simulink library "lib_controls"  (Simulink 7.9)
settings: Solver=ode45  SolverMode=SingleTasking  StartTime=0.0  StopTime=10.0  RelTol=1e-3
undefined symbols (not defined in the file): amb_tmp, cs_charge_deplete_bool, cs_charge_pwr, cs_charge_trq, cs_clt_tmp, cs_decel_fc_off, cs_decel_regen_threshold, cs_dl_assist_trq_threshold, cs_dl_regen_trq_threshold, cs_electric_decel_spd, cs_electric_launch_spd, cs_electric_launch_spd_hi, cs_electric_launch_spd_lo, cs_eng_min_spd, cs_eng_on_soc, cs_fc_init_state, cs_fc_max_pwr_frac, cs_fc_min_pwr_frac, cs_fc_on, cs_fc_pwr_opt, cs_fc_spd_opt, cs_fuzzy_fuel_mode, cs_hi_soc, cs_hi_trq_frac, cs_lo_soc, cs_lo_trq_frac, cs_max_gc_spd, cs_max_pwr, cs_max_pwr_fall_rate, cs_max_pwr_rise_rate, cs_mc_assist_max_frac, cs_mc_assist_min_frac, cs_mc_assist_slope, cs_mc_regen_max_frac, cs_mc_regen_min_frac, cs_mc_regen_slope, cs_mean_eff, cs_mean_eff_bool, cs_min_gc_spd, cs_min_off_time, cs_min_pwr, cs_min_trq_frac, cs_mph_avg_time, cs_off_trq_frac, cs_plot_output, cs_pwr, cs_regen_avg_time, cs_scale_factor, cs_shutoff, cs_soc_range, cs_spd, cs_target_soc, cs_trq_to_soc_factor, cvt_locus_pwr, cvt_locus_spd, cyc_mph, enable_sim_stop_distance, enable_sim_stop_max_spd, enable_sim_stop_speed, enable_sim_stop_time ... (+110)
libraries: lib_controls x124, simulink3 x18, lib_etc x1
(part 16 of 17)

== system lib_controls/<vc> par auto/gearbox control for use w/ AT/shifting1/time since last shift ==
  in_1 : Inport
  just shifted : Subsystem
      mask Display: disp('just\nshifted')
  timer : Subsystem
      mask Display: disp('timer')
  out_1 : Outport  InitialOutput=0
  wires:
  in_1/1 -> just shifted/1(in_1)
  just shifted/1(out_1) -> timer/1(trigger)
  timer/1(time) -> out_1/1

== system lib_controls/<vc> par auto/gearbox control for use w/ AT/upshift  command/load fraction ==
  In1 : Inport
  S-Function : S-Function  FunctionName=sfun_gearbox  Parameters=load, spd  EnableBusSupport=off
  Out1 : Outport  InitialOutput=0
  wires:
  S-Function/1 -> Out1/1
  In1/1 -> S-Function/1

== system lib_controls/<vc> par auto/parallel clutch control/gearbox speed estimator/Block NOTES ==
  note: The requested engine speed is replaced by an estimate of the
      | engine's previous speed whenever the vehicle missed the trace
      |  by more than 1 mph on the last time step.

== system lib_controls/<vc> par auto/parallel clutch control/gearbox speed estimator/dt ==
  Clock : Clock
  Memory1 : Memory  X0=-1
  Sum4 : Sum  Inputs=+-  SaturateOnIntegerOverflow=on  InputSameDT=on  OutDataTypeStr=Inherit: Same as first input
  Out1 : Outport  InitialOutput=0
  wires:
  Clock/1 -> Sum4/1, Memory1/1
  Memory1/1 -> Sum4/2
  Sum4/1 -> Out1/1

== system lib_controls/<vc> par auto s/a/gearbox control for use w/ AT  in parallel sa/downshift  command/load fraction ==
  In1 : Inport
  S-Function : S-Function  FunctionName=sfun_gearbox  Parameters=load, spd  EnableBusSupport=off
  Out1 : Outport  InitialOutput=0
  wires:
  S-Function/1 -> Out1/1
  In1/1 -> S-Function/1

== system lib_controls/<vc> par auto s/a/gearbox control for use w/ AT  in parallel sa/downshift  command1/load fraction ==
  In1 : Inport
  S-Function : S-Function  FunctionName=sfun_gearbox  Parameters=load, spd  EnableBusSupport=off
  Out1 : Outport  InitialOutput=0
  wires:
  In1/1 -> S-Function/1
  S-Function/1 -> Out1/1

== system lib_controls/<vc> par auto s/a/gearbox control for use w/ AT  in parallel sa/est. engine trq and spd/Block NOTES ==
  note: Estimate engine torque and speed associated with the previous gear, assuming that
      | the gearbox efficiency is constant.

== system lib_controls/<vc> par auto s/a/gearbox control for use w/ AT  in parallel sa/est. engine trq and spd/K_adv ==
  "Req'd output trq and spd (Nm), (rad/s)" : Inport
  K_adv=wout/(Tout)^0.5 : Fcn  Expr=u[2]/u[1]^0.5
  Saturation : Saturate  UpperLimit=max(htc_k_adv)  LowerLimit=min(htc_k_adv)
  Saturation2 : Saturate  UpperLimit=inf  LowerLimit=eps
  K_adv : Outport
  wires:
  "Req'd output trq and spd (Nm), (rad/s)"/1 -> Saturation2/1
  Saturation2/1 -> K_adv=wout/(Tout)^0.5/1
  K_adv=wout/(Tout)^0.5/1 -> Saturation/1
  Saturation/1 -> K_adv/1

== system lib_controls/<vc> par auto s/a/gearbox control for use w/ AT  in parallel sa/est. engine trq and spd assuming lockup/Block NOTES ==
  note: Estimate engine torque and speed associated with the current gear, assuming that
      | the gearbox efficiency is constant.

== system lib_controls/<vc> par auto s/a/gearbox control for use w/ AT  in parallel sa/shifting1/time since last shift ==
  in_1 : Inport
  just shifted : Subsystem
      mask Display: disp('just\nshifted')
  timer : Subsystem
      mask Display: disp('timer')
  out_1 : Outport  InitialOutput=0
  wires:
  in_1/1 -> just shifted/1(in_1)
  just shifted/1(out_1) -> timer/1(trigger)
  timer/1(time) -> out_1/1

== system lib_controls/<vc> par auto s/a/gearbox control for use w/ AT  in parallel sa/upshift  command/load fraction ==
  In1 : Inport
  S-Function : S-Function  FunctionName=sfun_gearbox  Parameters=load, spd  EnableBusSupport=off
  Out1 : Outport  InitialOutput=0
  wires:
  S-Function/1 -> Out1/1
  In1/1 -> S-Function/1

== system lib_controls/<vc> par balanced/parallel clutch control/gearbox speed estimator/Block NOTES ==
  note: The requested engine speed is replaced by an estimate of the
      | engine's previous speed whenever the vehicle missed the trace
      |  by more than 1 mph on the last time step.

== system lib_controls/<vc> par balanced/parallel clutch control/gearbox speed estimator/dt ==
  Clock : Clock
  Memory1 : Memory  X0=-1
  Sum4 : Sum  Inputs=+-  SaturateOnIntegerOverflow=on  InputSameDT=on  OutDataTypeStr=Inherit: Same as first input
  Out1 : Outport  InitialOutput=0
  wires:
  Clock/1 -> Sum4/1, Memory1/1
  Memory1/1 -> Sum4/2
  Sum4/1 -> Out1/1

== system lib_controls/<vc> par balanced/pre-TX parallel gearbox control/allow upshift?/Block NOTES1 ==
  note: This block prevents an upshift if it the engine is not on and
      | the upshift would make the motor power low enough that it
      | could not provide the required input power.  However, an upshift
      | is allowed if to stay in the current gear would put the motor
      | beyond 95% of its maximum speed.
      |
      | This block is to be used in pretransmission parallel hybrids
      | (where the engine and motor torques are combined on the
      | engine side of the transmission) ONLY.

== system lib_controls/<vc> par balanced/pre-TX parallel gearbox control/downshift  command/load fraction ==
  In1 : Inport
  S-Function : S-Function  FunctionName=sfun_gearbox  Parameters=load, spd  EnableBusSupport=off
  Out1 : Outport  InitialOutput=0
  wires:
  In1/1 -> S-Function/1
  S-Function/1 -> Out1/1

== system lib_controls/<vc> par balanced/pre-TX parallel gearbox control/gearbox speed estimator/Block NOTES ==
  note: The requested engine speed is replaced by an estimate of the
      | engine's previous speed whenever the vehicle missed the trace
      |  by more than 1 mph on the last time step.

== system lib_controls/<vc> par balanced/pre-TX parallel gearbox control/gearbox speed estimator/dt ==
  Clock : Clock
  Memory1 : Memory  X0=-1
  Sum4 : Sum  Inputs=+-  SaturateOnIntegerOverflow=on  InputSameDT=on  OutDataTypeStr=Inherit: Same as first input
  Out1 : Outport  InitialOutput=0
  wires:
  Clock/1 -> Sum4/1, Memory1/1
  Memory1/1 -> Sum4/2
  Sum4/1 -> Out1/1

== system lib_controls/<vc> par balanced/pre-TX parallel gearbox control/shifting1/time since last shift ==
  in_1 : Inport
  just shifted : Subsystem
      mask Display: disp('just\nshifted')
  timer : Subsystem
      mask Display: disp('timer')
  out_1 : Outport  InitialOutput=0
  wires:
  in_1/1 -> just shifted/1(in_1)
  just shifted/1(out_1) -> timer/1(trigger)
  timer/1(time) -> out_1/1

== system lib_controls/<vc> par balanced/pre-TX parallel gearbox control/upshift  command/load fraction ==
  In1 : Inport
  S-Function : S-Function  FunctionName=sfun_gearbox  Parameters=load, spd  EnableBusSupport=off
  Out1 : Outport  InitialOutput=0
  wires:
  In1/1 -> S-Function/1
  S-Function/1 -> Out1/1

== system lib_controls/<vc> par cvt/cvt control/Mode Selector/Block NOTES ==
  note: This block determines the operating mode of the parallel
      | hybrid vehicle equipped with a CVT:
      | Mode 1: motor only regen
      | if trq request is negative
      | Mode 2: motor only driving
      | if soc is greater than lo soc
      | and
      | pwr req is less than min engine pwr frac
      | Mode3: engine primary with motor assist
      | if pwr request between min and max pwr fractions
      | or
      | if soc less than low soc
      | Mode4: engine and motor combined system
      | if pwr req greater than max engine pwr frac

== system lib_controls/<vc> par cvt/parallel clutch control/gearbox speed estimator/Block NOTES ==
  note: The requested engine speed is replaced by an estimate of the
      | engine's previous speed whenever the vehicle missed the trace
      |  by more than 1 mph on the last time step.

== system lib_controls/<vc> par cvt/parallel clutch control/gearbox speed estimator/dt ==
  Clock : Clock
  Memory1 : Memory  X0=-1
  Sum4 : Sum  Inputs=+-  SaturateOnIntegerOverflow=on  InputSameDT=on  OutDataTypeStr=Inherit: Same as first input
  Out1 : Outport  InitialOutput=0
  wires:
  Sum4/1 -> Out1/1
  Memory1/1 -> Sum4/2
  Clock/1 -> Memory1/1, Sum4/1

== system lib_controls/<vc> prius/Coordinated  Controller/max engine efficiency point/Max fc spd (rad/s) ==
  mc spd : Inport
  <fc max rpm : Saturate  UpperLimit=4000*2*pi/60  LowerLimit=0
  f(gc max spd,veh spd) : Fcn  Expr=tx_pg_r/(tx_pg_r + tx_pg_s)*u + tx_pg_s/(tx_pg_r + tx_pg_s)*cs_max_gc_spd
  Max fc spd rad/s : Outport  InitialOutput=0
  wires:
  <fc max rpm/1 -> Max fc spd rad/s/1
  mc spd/1 -> f(gc max spd,veh spd)/1
  f(gc max spd,veh spd)/1 -> <fc max rpm/1

== system lib_controls/<vc> prius/Coordinated  Controller/max engine efficiency point/Min fc spd(rad/s) ==
  mc spd : Inport
  Constant2 : Constant  Value=vc_idle_spd
  Constant3 : Constant  Value=0
  MinMax1 : MinMax  Function=max  Inputs=2  SaturateOnIntegerOverflow=on  InputSameDT=on
  Switch2 : Switch  SaturateOnIntegerOverflow=on  InputSameDT=on
  To Workspace3 : ToWorkspace  VariableName=fc_min_spd  SampleTime=-1
  f(gc max spd,veh spd) : Fcn  Expr=tx_pg_r/(tx_pg_r + tx_pg_s)*u + tx_pg_s/(tx_pg_r + tx_pg_s)*cs_min_gc_spd
  min fc spd rad/s : Outport  InitialOutput=0
  wires:
  Switch2/1 -> To Workspace3/1, min fc spd rad/s/1
  Constant3/1 -> Switch2/3
  MinMax1/1 -> Switch2/1
  Constant2/1 -> MinMax1/1
  f(gc max spd,veh spd)/1 -> Switch2/2, MinMax1/2
  mc spd/1 -> f(gc max spd,veh spd)/1

== system lib_controls/<vc> prius/Coordinated  Controller/max engine efficiency point/at least  idle speed ==
  trq : Inport
  spd : Inport  Port=2
  Constant2 : Constant  Value=vc_idle_spd
  MinMax4 : MinMax  Function=max  Inputs=2  SaturateOnIntegerOverflow=on  InputSameDT=on
  Product : Product  SaturateOnIntegerOverflow=on  RndMeth=Zero  InputSameDT=on  OutDataTypeStr=Inherit: Same as first input
  Product1 : Product  Inputs=*/  SaturateOnIntegerOverflow=on  RndMeth=Zero  InputSameDT=on  OutDataTypeStr=Inherit: Same as first input
  Relational Operator : RelationalOperator  Operator=~=  InputSameDT=on
  Switch : Switch  Threshold=eps  SaturateOnIntegerOverflow=on  InputSameDT=on
  trq1 : Outport  InitialOutput=0
  spd1 : Outport  Port=2  InitialOutput=0
  wires:
  Product1/1 -> Switch/3
  Product/1 -> Product1/1
  trq/1 -> Product/1, Switch/1
  spd/1 -> Product/2, MinMax4/1
  Switch/1 -> trq1/1
  Relational Operator/1 -> Switch/2
  Constant2/1 -> Relational Operator/2, MinMax4/2
  MinMax4/1 -> Product1/2, spd1/1, Relational Operator/1

== system lib_controls/<vc> prius/Coordinated  Controller/max engine efficiency point/cranking? ==
  need engine on? : Inport
  constant : Constant  Value=cs_eng_min_spd
  constant1 : Constant  Value=cs_eng_min_spd
  logical  operator : Logic
  pwr : RelationalOperator  Operator=<  InputSameDT=on
  cranking? : Outport  InitialOutput=0
  wires:
  constant1/1 -> pwr/1
  constant/1 -> pwr/2
  pwr/1 -> logical  operator/2
  need engine on?/1 -> logical  operator/1
  logical  operator/1 -> cranking?/1

== system lib_controls/<vc> prius/Coordinated  Controller/max engine efficiency point/fuel on? ==
  cranking? : Inport
  need engine on?1 : Inport  Port=2
  logical  operator : Logic
  logical operator1 : Logic  Operator=NOT  Inputs=1
  "fuel on? " : Outport  InitialOutput=0
  wires:
  logical  operator/1 -> "fuel on? "/1
  cranking?/1 -> logical operator1/1
  need engine on?1/1 -> logical  operator/2
  logical operator1/1 -> logical  operator/1

== system lib_controls/<vc> prius/Coordinated  Controller/max engine efficiency point/max engine if pwr req>limit ==
  pwr req : Inport
  trq req : Inport  Port=2
  spd req : Inport  Port=3
  max fc spd : Inport  Port=4
  Switch3 : Switch  Threshold=25000  SaturateOnIntegerOverflow=on  InputSameDT=on
  Switch4 : Switch  Threshold=25000  SaturateOnIntegerOverflow=on  InputSameDT=on
  max_torque : Lookup  InputValues=fc_map_spd*fc_spd_scale  Table=fc_max_trq*fc_trq_scale  SaturateOnIntegerOverflow=on
  trq : Outport  InitialOutput=0
  spd : Outport  Port=2  InitialOutput=0
  wires:
  pwr req/1 -> Switch4/2, Switch3/2
  Switch4/1 -> spd/1
  Switch3/1 -> trq/1
  trq req/1 -> Switch3/3
  max_torque/1 -> Switch3/1
  max fc spd/1 -> max_torque/1, Switch4/1
  spd req/1 -> Switch4/3

== system lib_controls/<vc> prius/Coordinated  Controller/max engine efficiency point/need engine on? ==
  pwr requested : Inport
  0=Engine on 1=ZEV mode : Logic  Inputs=4
  SOC high enough? : Subsystem
  coolant temp high enough? : Subsystem
  has engine been off long enough? : Subsystem
  key_on : lib_controls/<vc> par/engine on (parallel hybrid)/key_on  MaskParam1=vc_key_on(:,1)  MaskParam2=vc_key_on(:,2)
  logical  operator : Logic  Inputs=3
  logical operator1 : Logic  Operator=NOT  Inputs=1
  pwr low enough? : Subsystem
  spd low enough? : Subsystem
  fc on=1 : Outport  InitialOutput=0
  wires:
  logical  operator/1 -> has engine been off long enough?/1(In1), fc on=1/1
  [fc_clt_tmp] -> coolant temp high enough?/1(In1)
  coolant temp high enough?/1(Out1) -> 0=Engine on 1=ZEV mode/4
  0=Engine on 1=ZEV mode/1 -> logical operator1/1
  SOC high enough?/1(Out1) -> 0=Engine on 1=ZEV mode/3
  [SOC] -> SOC high enough?/1(In1)
  [v_prev] -> spd low enough?/1(In1)
  pwr requested/1 -> pwr low enough?/1(In1)
  spd low enough?/1(Out1) -> 0=Engine on 1=ZEV mode/2
  pwr low enough?/1(Out1) -> 0=Engine on 1=ZEV mode/1
  has engine been off long enough?/1(Out1) -> logical  operator/3
  logical operator1/1 -> logical  operator/2
  key_on/1 -> logical  operator/1  "ignition key is on"

== system lib_controls/<vc> prius/Coordinated  Controller/max engine efficiency point/spd opt ==
  pwr req : Inport
  Product2 : Product  Inputs=**  SaturateOnIntegerOverflow=on  RndMeth=Zero  InputSameDT=on  OutDataTypeStr=Inherit: Same as first input
  Sum : Sum  SaturateOnIntegerOverflow=on  InputSameDT=on  OutDataTypeStr=Inherit: Same as first input
  effect of inertia  guess (Nm) : Subsystem
  fc spd opt : Lookup  InputValues=cs_fc_pwr_opt  Table=cs_fc_spd_opt  SaturateOnIntegerOverflow=on
  fc spd opt1 : Lookup  InputValues=cs_fc_pwr_opt  Table=cs_fc_spd_opt  SaturateOnIntegerOverflow=on
  spd opt : Outport  InitialOutput=0
  tag scope: inertia_effect_fc_guess=global
  wires:
  effect of inertia  guess (Nm)/1((Nm)) -> [inertia_effect_fc_guess], Product2/2
  pwr req/1 -> Sum/1, fc spd opt/1
  Product2/1 -> Sum/2
  Sum/1 -> fc spd opt1/1
  fc spd opt1/1 -> spd opt/1
  [fc_spd_prev] -> effect of inertia  guess (Nm)/2(prev spd)
  fc spd opt/1 -> Product2/1, effect of inertia  guess (Nm)/1(req'd spd (rad/s))

== system lib_controls/<vc> series/gearbox control for series  HV and EV/downshift  command/load fraction ==
  In1 : Inport
  S-Function : S-Function  FunctionName=sfun_gearbox  Parameters=load, spd  EnableBusSupport=off
  Out1 : Outport  InitialOutput=0
  wires:
  In1/1 -> S-Function/1
  S-Function/1 -> Out1/1

== system lib_controls/<vc> series/gearbox control for series  HV and EV/gearbox speed estimator/Block NOTES ==
  note: The requested motor speed is replaced by an estimate of the
      | engine's previous speed whenever the vehicle missed the trace
      |  by more than 1 mph on the last time step.

== system lib_controls/<vc> series/gearbox control for series  HV and EV/gearbox speed estimator/dt ==
  Clock : Clock
  Memory1 : Memory  X0=-1
  Sum4 : Sum  Inputs=+-  SaturateOnIntegerOverflow=on  InputSameDT=on  OutDataTypeStr=Inherit: Same as first input
  Out1 : Outport  InitialOutput=0
  wires:
  Sum4/1 -> Out1/1
  Memory1/1 -> Sum4/2
  Clock/1 -> Memory1/1, Sum4/1

== system lib_controls/<vc> series/gearbox control for series  HV and EV/shifting1/time since last shift ==
  in_1 : Inport
  just shifted : Subsystem
      mask Display: disp('just\nshifted')
  timer : Subsystem
      mask Display: disp('timer')
  out_1 : Outport  InitialOutput=0
  wires:
  in_1/1 -> just shifted/1(in_1)
  just shifted/1(out_1) -> timer/1(trigger)
  timer/1(time) -> out_1/1

== system lib_controls/<vc> series/gearbox control for series  HV and EV/upshift  command/load fraction ==
  In1 : Inport
  S-Function : S-Function  FunctionName=sfun_gearbox  Parameters=load, spd  EnableBusSupport=off
  Out1 : Outport  InitialOutput=0
  wires:
  In1/1 -> S-Function/1
  S-Function/1 -> Out1/1

== system lib_controls/Adaptive control strategy <cs>/Finds operation  point - energy/emissions  weighting/Minimize the  energy used  and emissions/Min. Energy/emis ==
  Treq : Inport
  wreq : Inport  Port=2
  DeltaSOC regen : Inport  Port=3
  SOC : Inport  Port=4
  cyc_mph_r : Inport  Port=5
  fc_clt_tmp : Inport  Port=6
  ex_cat_tmp : Inport  Port=7
  ess_tmp : Inport  Port=8
  Elect Aux  Load Power : Inport  Port=9
  Enable : EnablePort
  >0 : Saturate  UpperLimit=inf  LowerLimit=0
  CO temp eff : Lookup  InputValues=ex_cat_tmp_range  Table=ex_cat_co_frac  SaturateOnIntegerOverflow=on
  Demux : Demux  Outputs=2
  HC temp eff : Lookup  InputValues=ex_cat_tmp_range  Table=ex_cat_hc_frac  SaturateOnIntegerOverflow=on
  Mux2 : Mux  Inputs=14
  NOx temp eff : Lookup  InputValues=ex_cat_tmp_range  Table=ex_cat_nox_frac  SaturateOnIntegerOverflow=on
  PM temp eff : Lookup  InputValues=ex_cat_tmp_range  Table=ex_cat_pm_frac  SaturateOnIntegerOverflow=on
  S-Function : S-Function  FunctionName=minimum_energy9  Parameters=tc_mc_to_fc_ratio,fc_map_spd,fc_map_trq,fc_max_trq,fc_fuel_map,fc_nox_map,fc_pm_map,fc_hc_map,fc_co_map,fc_fuel_lhv,fc_fuel_den,fc_trq_scale,fc_spd_scale,ex_cat_lim,K_Energy,K_Emis,mpg_desired,hc_desired,co_desired,nox_desired,pm_desired,mc_max_trq,mc_map_spd,mc_map_trq,mc_eff_map,mc_trq_scale,mc_spd_scale,fc_eff_map  EnableBusSupport=off
  Scale Factor : Lookup  InputValues=cs_soc_range  Table=cs_scale_factor  SaturateOnIntegerOverflow=on
  "Tinit motor, (limited by max Tmotor and ess) and dT" : Subsystem
  lambda (non-negative) : Fcn  Expr=(fc_tstat-u)/(fc_tstat-20)
  limit Treq : Subsystem
  Tfc : Outport  OutputWhenDisabled=reset  InitialOutput=0
  Impact : Outport  Port=2  OutputWhenDisabled=reset  InitialOutput=0
  wires:
  Mux2/1 -> S-Function/1
  lambda (non-negative)/1 -> >0/1
  SOC/1 -> "Tinit motor, (limited by max Tmotor and ess) and dT"/3(SOC), Mux2/6, Scale Factor/1
  DeltaSOC regen/1 -> Mux2/5
  ex_cat_tmp/1 -> PM temp eff/1, NOx temp eff/1, HC temp eff/1, CO temp eff/1
  fc_clt_tmp/1 -> lambda (non-negative)/1
  wreq/1 -> Mux2/4, limit Treq/2(wreq), "Tinit motor, (limited by max Tmotor and ess) and dT"/2(wreq)
  limit Treq/1(Treq) -> Mux2/3, "Tinit motor, (limited by max Tmotor and ess) and dT"/1("Treq ")
  Treq/1 -> limit Treq/1("Treq ")
  "Tinit motor, (limited by max Tmotor and ess) and dT"/2(dT) -> Mux2/2
  "Tinit motor, (limited by max Tmotor and ess) and dT"/1(Tinit motor) -> Mux2/1
  HC temp eff/1 -> Mux2/7
  CO temp eff/1 -> Mux2/8
  NOx temp eff/1 -> Mux2/9
  PM temp eff/1 -> Mux2/10
  ess_tmp/1 -> "Tinit motor, (limited by max Tmotor and ess) and dT"/4(Tess), Mux2/14
  Scale Factor/1 -> Mux2/13
  >0/1 -> Mux2/12
  cyc_mph_r/1 -> Mux2/11
  S-Function/1 -> Demux/1
  Demux/2 -> Impact/1
  Demux/1 -> Tfc/1
  Elect Aux  Load Power/1 -> "Tinit motor, (limited by max Tmotor and ess) and dT"/5("Electrical Aux Loads (Power, W)")

== system lib_controls/Adaptive control strategy <cs>/Finds operation  point - energy/emissions  weighting/Minimize the  energy used  and emissions/Zero T/w/spd case ==
  Treq : Inport
  wreq : Inport  Port=2
  " " : Constant  Value=0
  " 2" : Constant  Value=0
  Logical Operator : Logic  Operator=OR
  Relational Operator : RelationalOperator  Operator===  InputSameDT=on
  Relational Operator1 : RelationalOperator  Operator===  InputSameDT=on
  zero req flag : Outport
  wires:
  " 2"/1 -> Relational Operator1/2
  Logical Operator/1 -> zero req flag/1
  wreq/1 -> Relational Operator/1
  Treq/1 -> Relational Operator1/1
  Relational Operator/1 -> Logical Operator/2
  Relational Operator1/1 -> Logical Operator/1
  " "/1 -> Relational Operator/2

== system lib_controls/SubSystem/front and rear brake controller (achievable)/braking force supplied by front friction brakes (N)/Block NOTES ==
  note: The variable "wh_max_front_fric_brake_force_N" must be assigned a positive value.
  note: If all braking was intended to be done by the drivetrain, the front friction brakes will do 60% of the braking.
  note: where the denominator can also be expressed as [1 - front_axle_drivetrain_brake_fraction(vehicle speed)].
  note: [front_axle_friction_brake_fraction(vehicle speed)]
      | ------------------------------------------------------------------------------
      | [front_axle_friction_brake_fraction(vehicle speed) + rear_axle_friction_brake_fraction(vehicle speed)]
  note: If additional braking force is required to meet the specified deceleration, input #1 will be negative.
      | The fraction of the additional req'd braking force made up by the front-axle friction brakes is given by:

== system lib_controls/SubSystem/shifting/time since last shift/just shifted ==
  in_1 : Inport
  Memory : Memory  X0=1
  Relational Operator : RelationalOperator  Operator=~=  InputSameDT=on
  out_1 : Outport  InitialOutput=0
  wires:
  Relational Operator/1 -> out_1/1
  Memory/1 -> Relational Operator/1
  in_1/1 -> Relational Operator/2, Memory/1

== system lib_controls/SubSystem/shifting/time since last shift/timer ==
  trigger : Inport
  Constant : Constant
  Constant1 : Constant  Value=0
  Constant2 : Constant  Value=0
  Switch : Switch  Threshold=eps  SaturateOnIntegerOverflow=on  InputSameDT=on
  no-lag Reset Integrator : Subsystem  mask(No-lag Reset Integrator){initval=15}
      mask prompts: initval "Initial Value"
      mask help: No-lag Reset Integrator
      mask Help: Integrates first input using Euler technique.\nAt the time step that input 2 <> zero,\noutput is reset to input 3.
      mask Display: disp('1/s\nw/ reset\nno lag')
  time : Outport  InitialOutput=0
  wires:
  Switch/1 -> time/1
  trigger/1 -> Switch/2, no-lag Reset Integrator/2(in_2)
  Constant2/1 -> Switch/1
  Constant/1 -> no-lag Reset Integrator/1(in_1)
  Constant1/1 -> no-lag Reset Integrator/3(in_3)
  no-lag Reset Integrator/1(out_1) -> Switch/3

== system lib_controls/SubSystem/sim stop subsystem/stop sim max spd/Block NOTES ==
  note: When enabled, stop the simulation when the current speed is greater
      | than zero and is less than or equal to the speed at gb_shift_delay*5+1
      | seconds ago (i.e. vehicle has reached a constant max speed). Only used
      | during acceleration test.

== system lib_controls/SubSystem/traction control/apply tire traction limit to req'd speed (m/s)/Block NOTES ==
  note: This block limits the requested speed by the maximum and minimum attainable given the maximum traction of the tires.
      | That is, acceleration and braking maneuvers are limited to the point of imminent skidding.
  note: The above equations are derived by solving F_maxaccel=mass*a_max for the maximum or minimum speed at the end of the time step,
      | given that F_maxaccel depends on the weight borne by the front tires which in turn depends on the vehicle's acceleration rate.
  note: Front-wheel drive is assumed, and weight transfer due to acceleration is included in the calculation of maximum tractive force.

== system lib_controls/SubSystem/traction control/apply tire traction limit to req'd speed (m/s)/max speed at END of time step given tire traction limit (m/s) ==
  in_1 : Inport
  in_2 : Inport  Port=2
  Fcn : Fcn  Expr=1/u
  Product : Product  SaturateOnIntegerOverflow=on  RndMeth=Zero  InputSameDT=on  OutDataTypeStr=Inherit: Same as first input
  out_1 : Outport  InitialOutput=0
  wires:
  in_2/1 -> Fcn/1
  Product/1 -> out_1/1
  Fcn/1 -> Product/2
  in_1/1 -> Product/1

== system lib_controls/SubSystem/traction control/apply tire traction limit to req'd speed (m/s)/min speed at END of time step given tire traction limit (m/s) ==
  in_1 : Inport
  in_2 : Inport  Port=2
  Fcn : Fcn  Expr=1/u
  Product : Product  SaturateOnIntegerOverflow=on  RndMeth=Zero  InputSameDT=on  OutDataTypeStr=Inherit: Same as first input
  out_1 : Outport  InitialOutput=0
  wires:
  in_1/1 -> Product/1
  Fcn/1 -> Product/2
  Product/1 -> out_1/1
  in_2/1 -> Fcn/1

== system lib_controls/SubSystem/traction control/enforce max.  front axle tractive force  due to slip (N)/Block NOTES ==
  note: No more force will be requested of the drivetrain than can be transmitted by the front tires.
      | This transmittable force is computed taking into account the slip characteristics of the tires
      | and the variable, acceleration-dependent weight borne by the front axle.

== system lib_controls/SubSystem/traction control 2 axle/apply tire traction limit to req'd speed (m/s)/Block NOTES ==
  note: This block limits the requested speed by the maximum and minimum attainable given the maximum traction of the tires.
      | That is, acceleration and braking maneuvers are limited to the point of imminent skidding.
  note: The above equations are derived by solving F_maxaccel=mass*a_max for the maximum or minimum speed at the end of the time step,
      | given that F_maxaccel depends on the weight borne by the front tires which in turn depends on the vehicle's acceleration rate.
  note: Front-wheel drive is assumed, and weight transfer due to acceleration is included in the calculation of maximum tractive force.

== system lib_controls/SubSystem/traction control 2 axle/apply tire traction limit to req'd speed (m/s)/max speed at END of time step given tire traction limit (m/s) ==
  in_1 : Inport
  in_2 : Inport  Port=2
  Fcn : Fcn  Expr=1/u
  Product : Product  SaturateOnIntegerOverflow=on  RndMeth=Zero  InputSameDT=on  OutDataTypeStr=Inherit: Same as first input
  out_1 : Outport  InitialOutput=0
  wires:
  in_1/1 -> Product/1
  Fcn/1 -> Product/2
  Product/1 -> out_1/1
  in_2/1 -> Fcn/1

== system lib_controls/SubSystem/traction control 2 axle/apply tire traction limit to req'd speed (m/s)/min speed at END of time step given tire traction limit (m/s) ==
  in_1 : Inport
  in_2 : Inport  Port=2
  Fcn : Fcn  Expr=1/u
  Product : Product  SaturateOnIntegerOverflow=on  RndMeth=Zero  InputSameDT=on  OutDataTypeStr=Inherit: Same as first input
  out_1 : Outport  InitialOutput=0
  wires:
  in_2/1 -> Fcn/1
  Product/1 -> out_1/1
  Fcn/1 -> Product/2
  in_1/1 -> Product/1

== system lib_controls/SubSystem/traction control 2 axle/apply tire traction limit to req'd speed (m/s)/rear slip terms ==
  initial speed : Inport
  1/dt : Inport  Port=2
  sin(theta) : Inport  Port=3
  Constant12 : Constant  Value=max(wh_slip_force_coeff)*(-1*veh_cg_height)/veh_wheelbase
  Constant8 : Constant  Value=veh_gravity
  Product13 : Product  Inputs=3  SaturateOnIntegerOverflow=on  RndMeth=Zero  InputSameDT=on  OutDataTypeStr=Inherit: Same as first input
  Product14 : Product  Inputs=4  SaturateOnIntegerOverflow=on  RndMeth=Zero  InputSameDT=on  OutDataTypeStr=Inherit: Same as first input
  current  veh mass (kg) : lib_controls/SubSystem/current veh mass (kg)
      settings: RTWFcnNameOpts=Auto  RTWFileNameOpts=Auto
  Out1 : Outport
  Out2 : Outport  Port=2
  wires:
  sin(theta)/1 -> Product13/3
  Product13/1 -> Out2/1
  1/dt/1 -> Product14/3
  Product14/1 -> Out1/1
  initial speed/1 -> Product14/2
  current  veh mass (kg)/1 -> Product14/4
  Constant8/1 -> Product13/2
  Constant12/1 -> Product13/1, Product14/1

== system lib_controls/SubSystem/traction control 2 axle/enforce max.  front axle tractive force  due to slip (N)/Block NOTES ==
  note: No more force will be requested of the drivetrain than can be transmitted by the front tires.
      | This transmittable force is computed taking into account the slip characteristics of the tires
      | and the variable, acceleration-dependent weight borne by the front axle.

== system lib_controls/SubSystem/traction control 2 axle/enforce max.  front axle tractive force  due to slip (N)/front ==
  In1 : Inport
  In2 : Inport  Port=2
  Clock : Clock
  Constant : Constant  Value=veh_cg_height/veh_wheelbase
  Constant1 : Constant  Value=veh_gravity*veh_front_wt_frac
  Gain1 : Gain  Gain=2  SaturateOnIntegerOverflow=on  OutDataTypeStr=Inherit: Same as input  ParamDataTypeStr=Inherit: Same as input
  Gain2 : Gain  Gain=veh_gravity  SaturateOnIntegerOverflow=on  OutDataTypeStr=Inherit: Same as input  ParamDataTypeStr=Inherit: Same as input
  Memory1 : Memory  X0=-0.1
  Product : Product  Inputs=*/  SaturateOnIntegerOverflow=on  RndMeth=Zero  InputSameDT=on  OutDataTypeStr=Inherit: Same as first input
  Product1 : Product  Inputs=3  SaturateOnIntegerOverflow=on  RndMeth=Zero  InputSameDT=on  OutDataTypeStr=Inherit: Same as first input
  Product3 : Product  Inputs=3  SaturateOnIntegerOverflow=on  RndMeth=Zero  InputSameDT=on  OutDataTypeStr=Inherit: Same as first input
  Sum : Sum  Inputs=+-  SaturateOnIntegerOverflow=on  InputSameDT=on  OutDataTypeStr=Inherit: Same as first input
  Sum1 : Sum  Inputs=+-  SaturateOnIntegerOverflow=on  InputSameDT=on  OutDataTypeStr=Inherit: Same as first input
  Sum2 : Sum  SaturateOnIntegerOverflow=on  InputSameDT=on  OutDataTypeStr=Inherit: Same as first input
  Trig Fn : Trigonometry  Operator=atan
  Trig Fn1 : Trigonometry
  Trig Fn2 : Trigonometry  Operator=cos
  current veh mass (kg) : lib_controls/SubSystem/current veh mass (kg)
      settings: RTWFcnNameOpts=Auto  RTWFileNameOpts=Auto
  weight on front axle (N)1 : Sum  Inputs=-+  SaturateOnIntegerOverflow=on  InputSameDT=on  OutDataTypeStr=Inherit: Same as first input
  Out1 : Outport
  wires:
  weight on front axle (N)1/1 -> Out1/1
  In2/1 -> Sum/2
  In1/1 -> Sum/1
  current veh mass (kg)/1 -> Product3/1, Product1/3
  Trig Fn2/1 -> Product3/2
  Constant1/1 -> Product3/3
  Product3/1 -> weight on front axle (N)1/2
  Trig Fn/1 -> Trig Fn2/1, Trig Fn1/1
  Gain2/1 -> Sum2/2
  Trig Fn1/1 -> Gain2/1
  [grade] -> Trig Fn/1
  Sum2/1 -> Product1/2
  Gain1/1 -> Sum2/1
  Product/1 -> Gain1/1
  Sum1/1 -> Product/2
  Memory1/1 -> Sum1/2
  Clock/1 -> Memory1/1, Sum1/1
  Sum/1 -> Product/1
  Constant/1 -> Product1/1
  Product1/1 -> weight on front axle (N)1/1

== system lib_controls/SubSystem/traction control 2 axle/enforce max.  front axle tractive force  due to slip (N)/rear ==
  In1 : Inport
  In2 : Inport  Port=2
  Clock : Clock
  Constant : Constant  Value=(-1*veh_cg_height)/veh_wheelbase
  Constant1 : Constant  Value=veh_gravity*(1-veh_front_wt_frac)
  Gain1 : Gain  Gain=2  SaturateOnIntegerOverflow=on  OutDataTypeStr=Inherit: Same as input  ParamDataTypeStr=Inherit: Same as input
  Gain2 : Gain  Gain=veh_gravity  SaturateOnIntegerOverflow=on  OutDataTypeStr=Inherit: Same as input  ParamDataTypeStr=Inherit: Same as input
  Memory1 : Memory  X0=-0.1
  Product : Product  Inputs=*/  SaturateOnIntegerOverflow=on  RndMeth=Zero  InputSameDT=on  OutDataTypeStr=Inherit: Same as first input
  Product1 : Product  Inputs=3  SaturateOnIntegerOverflow=on  RndMeth=Zero  InputSameDT=on  OutDataTypeStr=Inherit: Same as first input
  Product3 : Product  Inputs=3  SaturateOnIntegerOverflow=on  RndMeth=Zero  InputSameDT=on  OutDataTypeStr=Inherit: Same as first input
  Sum : Sum  Inputs=+-  SaturateOnIntegerOverflow=on  InputSameDT=on  OutDataTypeStr=Inherit: Same as first input
  Sum1 : Sum  Inputs=+-  SaturateOnIntegerOverflow=on  InputSameDT=on  OutDataTypeStr=Inherit: Same as first input
  Sum2 : Sum  SaturateOnIntegerOverflow=on  InputSameDT=on  OutDataTypeStr=Inherit: Same as first input
  Trig Fn : Trigonometry  Operator=atan
  Trig Fn1 : Trigonometry
  Trig Fn2 : Trigonometry  Operator=cos
  current veh mass (kg) : lib_controls/SubSystem/current veh mass (kg)
      settings: RTWFcnNameOpts=Auto  RTWFileNameOpts=Auto
  weight on rear axle (N) : Sum  Inputs=-+  SaturateOnIntegerOverflow=on  InputSameDT=on  OutDataTypeStr=Inherit: Same as first input
  Out1 : Outport
  wires:
  weight on rear axle (N)/1 -> Out1/1
  In2/1 -> Sum/2
  In1/1 -> Sum/1
  current veh mass (kg)/1 -> Product3/1, Product1/3
  Trig Fn2/1 -> Product3/2
  Constant1/1 -> Product3/3
  Product3/1 -> weight on rear axle (N)/2
  Trig Fn/1 -> Trig Fn2/1, Trig Fn1/1
  Gain2/1 -> Sum2/2
  Trig Fn1/1 -> Gain2/1
  [grade] -> Trig Fn/1
  Sum2/1 -> Product1/2
  Gain1/1 -> Sum2/1
  Product/1 -> Gain1/1
  Sum1/1 -> Product/2
  Memory1/1 -> Sum1/2
  Clock/1 -> Memory1/1, Sum1/1
  Sum/1 -> Product/1
  Constant/1 -> Product1/1
  Product1/1 -> weight on rear axle (N)/1

== system lib_controls/SubSystem/traction control J2452/apply tire traction limit to req'd speed (m/s)/Block NOTES ==
  note: This block limits the requested speed by the maximum and minimum attainable given the maximum traction of the tires.
      | That is, acceleration and braking maneuvers are limited to the point of imminent skidding.
  note: The above equations are derived by solving F_maxaccel=mass*a_max for the maximum or minimum speed at the end of the time step,
      | given that F_maxaccel depends on the weight borne by the front tires which in turn depends on the vehicle's acceleration rate.
  note: Front-wheel drive is assumed, and weight transfer due to acceleration is included in the calculation of maximum tractive force.
      |
      | SAE J2452 rolling resistance model is included.
      |
      | Rolling resistance coefficients veh_rr_a and veh_rr_b have units of N/km/h and N/(km/h)^2 respectively.
      | Each is converted to N/m/s and N/(m/s)^2 with the gain blocks before it is input into the final traction equation.
      |
      | Veh_rr_a, veh_rr_b, and veh_rr_c must always be adjusted for roadwheel curvature before use.

== system lib_controls/SubSystem/traction control J2452/enforce max.  front axle tractive force  due to slip (N)/Block NOTES ==
  note: No more force will be requested of the drivetrain than can be transmitted by the front tires.
      | This transmittable force is computed taking into account the slip characteristics of the tires
      | and the variable, acceleration-dependent weight borne by the front axle.

== system lib_controls/SubSystem/traction control J2452 2 axle/apply tire traction limit to req'd speed (m/s)/Block NOTES ==
  note: This block limits the requested speed by the maximum and minimum attainable given the maximum traction of the tires.
      | That is, acceleration and braking maneuvers are limited to the point of imminent skidding.
  note: The above equations are derived by solving F_maxaccel=mass*a_max for the maximum or minimum speed at the end of the time step,
      | given that F_maxaccel depends on the weight borne by the front tires which in turn depends on the vehicle's acceleration rate.
  note: Front-wheel drive is assumed, and weight transfer due to acceleration is included in the calculation of maximum tractive force.
      |
      | SAE J2452 rolling resistance model is included.
      |
      | Rolling resistance coefficients veh_rr_a and veh_rr_b have units of N/km/h and N/(km/h)^2 respectively.
      | Each is converted to N/m/s and N/(m/s)^2 with the gain blocks before it is input into the final traction equation.
      |
      | Veh_rr_a, veh_rr_b, and veh_rr_c must always be adjusted for roadwheel curvature before use.

== system lib_controls/SubSystem/traction control J2452 2 axle/apply tire traction limit to req'd speed (m/s)/Subsystem ==
  Constant16 : Constant  Value=(-1*veh_cg_height/veh_wheelbase)
  Constant17 : Constant  Value=wh_radius
  Constant18 : Constant  Value=(1-veh_front_wt_frac)
  Constant19 : Constant  Value=0
  Error Check1 : MinMax  Function=max  Inputs=2  SaturateOnIntegerOverflow=on  InputSameDT=on
  Memory2 : Memory  X0=-0.1
  Product10 : Product  Inputs=3  SaturateOnIntegerOverflow=on  RndMeth=Zero  InputSameDT=on  OutDataTypeStr=Inherit: Same as first input
  Product11 : Product  SaturateOnIntegerOverflow=on  RndMeth=Zero  InputSameDT=on  OutDataTypeStr=Inherit: Same as first input
  Product12 : Product  SaturateOnIntegerOverflow=on  RndMeth=Zero  InputSameDT=on  OutDataTypeStr=Inherit: Same as first input
  Product13 : Product  SaturateOnIntegerOverflow=on  RndMeth=Zero  InputSameDT=on  OutDataTypeStr=Inherit: Same as first input
  Sum2 : Sum  Inputs=+-  SaturateOnIntegerOverflow=on  InputSameDT=on  OutDataTypeStr=Inherit: Same as first input
  Sum3 : Sum  Inputs=+-  SaturateOnIntegerOverflow=on  InputSameDT=on  OutDataTypeStr=Inherit: Same as first input
  Sum6 : Sum  Inputs=-+  SaturateOnIntegerOverflow=on  InputSameDT=on  OutDataTypeStr=Inherit: Same as first input
  Trig Fn7 : Trigonometry  Operator=atan
  Trig Fn8 : Trigonometry  Operator=cos
  current veh mass (kg)4 : lib_controls/SubSystem/current veh mass (kg)
      settings: RTWFcnNameOpts=Auto  RTWFileNameOpts=Auto
  Out1 : Outport
  Out2 : Outport  Port=2
  wires:
  Error Check1/1 -> Sum6/1, Out1/1  "Nf"
  Constant19/1 -> Error Check1/2
  Sum2/1 -> Error Check1/1  "Nf"
  Product13/1 -> Sum6/2  "W"
  Memory2/1 -> Product11/1
  [wh_trq_a] -> Memory2/1
  current veh mass (kg)4/1 -> Product13/2, Product10/3
  Constant18/1 -> Product10/2
  Trig Fn8/1 -> Product13/1, Product10/1
  Trig Fn7/1 -> Trig Fn8/1
  [grade] -> Trig Fn7/1
  Product10/1 -> Sum2/1
  Constant17/1 -> Product11/2
  Product11/1 -> Sum3/1
  [Fr_out] -> Sum3/2
  Sum3/1 -> Product12/1
  Constant16/1 -> Product12/2
  Product12/1 -> Sum2/2
  Sum6/1 -> Out2/1  "Nr=W-Nf"

== system lib_controls/SubSystem/traction control J2452 2 axle/apply tire traction limit to req'd speed (m/s)/Subsystem1 ==
  Constant15 : Constant  Value=max(wh_slip_force_coeff)*veh_gravity*(1-veh_front_wt_frac)
  Product8 : Product  Inputs=3  SaturateOnIntegerOverflow=on  RndMeth=Zero  InputSameDT=on  OutDataTypeStr=Inherit: Same as first input
  Trig Fn5 : Trigonometry  Operator=atan
  Trig Fn6 : Trigonometry  Operator=cos
  current veh mass (kg)3 : lib_controls/SubSystem/current veh mass (kg)
      settings: RTWFcnNameOpts=Auto  RTWFileNameOpts=Auto
  Out1 : Outport
  wires:
  Trig Fn6/1 -> Product8/2
  current veh mass (kg)3/1 -> Product8/3
  Constant15/1 -> Product8/1
  Trig Fn5/1 -> Trig Fn6/1
  [grade] -> Trig Fn5/1
  Product8/1 -> Out1/1  "Ftract"

== system lib_controls/fuel cell control strategy <cs>/FC on/no-lag Reset Integrator/dt ==
  Clock : Clock
  Memory1 : Memory  X0=-1
  Sum1 : Sum  Inputs=+-  SaturateOnIntegerOverflow=on  InputSameDT=on  OutDataTypeStr=Inherit: Same as first input
  out_1 : Outport  InitialOutput=0
  wires:
  Sum1/1 -> out_1/1
  Memory1/1 -> Sum1/2
  Clock/1 -> Memory1/1, Sum1/1

== system lib_controls/series hybrid control stategy  <cs>/FC on/no-lag Reset Integrator/dt ==
  Clock : Clock
  Memory1 : Memory  X0=-1
  Sum1 : Sum  Inputs=+-  SaturateOnIntegerOverflow=on  InputSameDT=on  OutDataTypeStr=Inherit: Same as first input
  out_1 : Outport  InitialOutput=0
  wires:
  Clock/1 -> Sum1/1, Memory1/1
  Memory1/1 -> Sum1/2
  Sum1/1 -> out_1/1

== system lib_controls/<vc> conv/gearbox  control/shifting1/time since last shift/just shifted ==
  in_1 : Inport
  Memory : Memory  X0=1
  Relational Operator : RelationalOperator  Operator=~=  InputSameDT=on
  out_1 : Outport  InitialOutput=0
  wires:
  in_1/1 -> Memory/1, Relational Operator/2
  Memory/1 -> Relational Operator/1
  Relational Operator/1 -> out_1/1

== system lib_controls/<vc> conv/gearbox  control/shifting1/time since last shift/timer ==
  trigger : Inport
  Constant : Constant
  Constant1 : Constant  Value=0
  Constant2 : Constant  Value=0
  Switch : Switch  Threshold=eps  SaturateOnIntegerOverflow=on  InputSameDT=on
  no-lag Reset Integrator : Subsystem  mask(No-lag Reset Integrator){initval=15}
      mask prompts: initval "Initial Value"
      mask help: No-lag Reset Integrator
      mask Help: Integrates first input using Euler technique.\nAt the time step that input 2 <> zero,\noutput is reset to input 3.
      mask Display: disp('1/s\nw/ reset\nno lag')
  time : Outport  InitialOutput=0
  wires:
  no-lag Reset Integrator/1(out_1) -> Switch/3
  Constant1/1 -> no-lag Reset Integrator/3(in_3)
  Constant/1 -> no-lag Reset Integrator/1(in_1)
  Constant2/1 -> Switch/1
  trigger/1 -> no-lag Reset Integrator/2(in_2), Switch/2
  Switch/1 -> time/1

== system lib_controls/<vc> conv Saber custom/gearbox  control/shifting1/time since last shift/just shifted ==
  in_1 : Inport
  Memory : Memory  X0=1
  Relational Operator : RelationalOperator  Operator=~=  InputSameDT=on
  out_1 : Outport  InitialOutput=0
  wires:
  Relational Operator/1 -> out_1/1
  Memory/1 -> Relational Operator/1
  in_1/1 -> Relational Operator/2, Memory/1

== system lib_controls/<vc> conv Saber custom/gearbox  control/shifting1/time since last shift/timer ==
  trigger : Inport
  Constant : Constant
  Constant1 : Constant  Value=0
  Constant2 : Constant  Value=0
  Switch : Switch  Threshold=eps  SaturateOnIntegerOverflow=on  InputSameDT=on
  no-lag Reset Integrator : Subsystem  mask(No-lag Reset Integrator){initval=15}
      mask prompts: initval "Initial Value"
      mask help: No-lag Reset Integrator
      mask Help: Integrates first input using Euler technique.\nAt the time step that input 2 <> zero,\noutput is reset to input 3.
      mask Display: disp('1/s\nw/ reset\nno lag')
  time : Outport  InitialOutput=0
  wires:
  Switch/1 -> time/1
  trigger/1 -> Switch/2, no-lag Reset Integrator/2(in_2)
  Constant2/1 -> Switch/1
  Constant/1 -> no-lag Reset Integrator/1(in_1)
  Constant1/1 -> no-lag Reset Integrator/3(in_3)
  no-lag Reset Integrator/1(out_1) -> Switch/3

== system lib_controls/<vc> conv auto/gearbox control for use w/ AT/shifting1/time since last shift/just shifted ==
  in_1 : Inport
  Memory : Memory  X0=1
  Relational Operator : RelationalOperator  Operator=~=  InputSameDT=on
  out_1 : Outport  InitialOutput=0
  wires:
  in_1/1 -> Memory/1, Relational Operator/2
  Memory/1 -> Relational Operator/1
  Relational Operator/1 -> out_1/1

== system lib_controls/<vc> conv auto/gearbox control for use w/ AT/shifting1/time since last shift/timer ==
  trigger : Inport
  Constant : Constant
  Constant1 : Constant  Value=0
  Constant2 : Constant  Value=0
  Switch : Switch  Threshold=eps  SaturateOnIntegerOverflow=on  InputSameDT=on
  no-lag Reset Integrator : Subsystem  mask(No-lag Reset Integrator){initval=15}
      mask prompts: initval "Initial Value"
      mask help: No-lag Reset Integrator
      mask Help: Integrates first input using Euler technique.\nAt the time step that input 2 <> zero,\noutput is reset to input 3.
      mask Display: disp('1/s\nw/ reset\nno lag')
  time : Outport  InitialOutput=0
  wires:
  no-lag Reset Integrator/1(out_1) -> Switch/3
  Constant1/1 -> no-lag Reset Integrator/3(in_3)
  Constant/1 -> no-lag Reset Integrator/1(in_1)
  Constant2/1 -> Switch/1
  trigger/1 -> no-lag Reset Integrator/2(in_2), Switch/2
  Switch/1 -> time/1

== system lib_controls/<vc> conv auto Saber custom/gearbox control for use w/ AT/shifting1/time since last shift/just shifted ==
  in_1 : Inport
  Memory : Memory  X0=1
  Relational Operator : RelationalOperator  Operator=~=  InputSameDT=on
  out_1 : Outport  InitialOutput=0
  wires:
  Relational Operator/1 -> out_1/1
  Memory/1 -> Relational Operator/1
  in_1/1 -> Relational Operator/2, Memory/1

== system lib_controls/<vc> conv auto Saber custom/gearbox control for use w/ AT/shifting1/time since last shift/timer ==
  trigger : Inport
  Constant : Constant
  Constant1 : Constant  Value=0
  Constant2 : Constant  Value=0
  Switch : Switch  Threshold=eps  SaturateOnIntegerOverflow=on  InputSameDT=on
  no-lag Reset Integrator : Subsystem  mask(No-lag Reset Integrator){initval=15}
      mask prompts: initval "Initial Value"
      mask help: No-lag Reset Integrator
      mask Help: Integrates first input using Euler technique.\nAt the time step that input 2 <> zero,\noutput is reset to input 3.
      mask Display: disp('1/s\nw/ reset\nno lag')
  time : Outport  InitialOutput=0
  wires:
  Switch/1 -> time/1
  trigger/1 -> Switch/2, no-lag Reset Integrator/2(in_2)
  Constant2/1 -> Switch/1
  Constant/1 -> no-lag Reset Integrator/1(in_1)
  Constant1/1 -> no-lag Reset Integrator/3(in_3)
  no-lag Reset Integrator/1(out_1) -> Switch/3

== system lib_controls/<vc> ev/gearbox control for series  HV and EV/shifting1/time since last shift/just shifted ==
  in_1 : Inport
  Memory : Memory  X0=1
  Relational Operator : RelationalOperator  Operator=~=  InputSameDT=on
  out_1 : Outport  InitialOutput=0
  wires:
  Relational Operator/1 -> out_1/1
  Memory/1 -> Relational Operator/1
  in_1/1 -> Relational Operator/2, Memory/1

== system lib_controls/<vc> ev/gearbox control for series  HV and EV/shifting1/time since last shift/timer ==
  trigger : Inport
  Constant : Constant
  Constant1 : Constant  Value=0
  Constant2 : Constant  Value=0
  Switch : Switch  Threshold=eps  SaturateOnIntegerOverflow=on  InputSameDT=on
  no-lag Reset Integrator : Subsystem  mask(No-lag Reset Integrator){initval=15}
      mask prompts: initval "Initial Value"
      mask help: No-lag Reset Integrator
      mask Help: Integrates first input using Euler technique.\nAt the time step that input 2 <> zero,\noutput is reset to input 3.
      mask Display: disp('1/s\nw/ reset\nno lag')
  time : Outport  InitialOutput=0
  wires:
  Switch/1 -> time/1
  trigger/1 -> Switch/2, no-lag Reset Integrator/2(in_2)
  Constant2/1 -> Switch/1
  Constant/1 -> no-lag Reset Integrator/1(in_1)
  Constant1/1 -> no-lag Reset Integrator/3(in_3)
  no-lag Reset Integrator/1(out_1) -> Switch/3

== system lib_controls/<vc> fuel cell/gearbox control for series  HV and EV/shifting1/time since last shift/just shifted ==
  in_1 : Inport
  Memory : Memory  X0=1
  Relational Operator : RelationalOperator  Operator=~=  InputSameDT=on
  out_1 : Outport  InitialOutput=0
  wires:
  Relational Operator/1 -> out_1/1
  Memory/1 -> Relational Operator/1
  in_1/1 -> Relational Operator/2, Memory/1

== system lib_controls/<vc> fuel cell/gearbox control for series  HV and EV/shifting1/time since last shift/timer ==
  trigger : Inport
  Constant : Constant
  Constant1 : Constant  Value=0
  Constant2 : Constant  Value=0
  Switch : Switch  Threshold=eps  SaturateOnIntegerOverflow=on  InputSameDT=on
  no-lag Reset Integrator : Subsystem  mask(No-lag Reset Integrator){initval=15}
      mask prompts: initval "Initial Value"
      mask help: No-lag Reset Integrator
      mask Help: Integrates first input using Euler technique.\nAt the time step that input 2 <> zero,\noutput is reset to input 3.
      mask Display: disp('1/s\nw/ reset\nno lag')
  time : Outport  InitialOutput=0
  wires:
  Switch/1 -> time/1
  trigger/1 -> Switch/2, no-lag Reset Integrator/2(in_2)
  Constant2/1 -> Switch/1
  Constant/1 -> no-lag Reset Integrator/1(in_1)
  Constant1/1 -> no-lag Reset Integrator/3(in_3)
  no-lag Reset Integrator/1(out_1) -> Switch/3

== system lib_controls/<vc> insight/pre-TX parallel gearbox control/shifting1/time since last shift/just shifted ==
  in_1 : Inport
  Memory : Memory  X0=1
  Relational Operator : RelationalOperator  Operator=~=  InputSameDT=on
  out_1 : Outport  InitialOutput=0
  wires:
  in_1/1 -> Memory/1, Relational Operator/2
  Memory/1 -> Relational Operator/1
  Relational Operator/1 -> out_1/1

== system lib_controls/<vc> insight/pre-TX parallel gearbox control/shifting1/time since last shift/timer ==
  trigger : Inport
  Constant : Constant
  Constant1 : Constant  Value=0
  Constant2 : Constant  Value=0
  Switch : Switch  Threshold=eps  SaturateOnIntegerOverflow=on  InputSameDT=on
  no-lag Reset Integrator : Subsystem  mask(No-lag Reset Integrator){initval=15}
      mask prompts: initval "Initial Value"
      mask help: No-lag Reset Integrator
      mask Help: Integrates first input using Euler technique.\nAt the time step that input 2 <> zero,\noutput is reset to input 3.
      mask Display: disp('1/s\nw/ reset\nno lag')
  time : Outport  InitialOutput=0
  wires:
  no-lag Reset Integrator/1(out_1) -> Switch/3
  Constant1/1 -> no-lag Reset Integrator/3(in_3)
  Constant/1 -> no-lag Reset Integrator/1(in_1)
  Constant2/1 -> Switch/1
  trigger/1 -> no-lag Reset Integrator/2(in_2), Switch/2
  Switch/1 -> time/1

== system lib_controls/<vc> par/pre-TX parallel gearbox control/shifting1/time since last shift/just shifted ==
  in_1 : Inport
  Memory : Memory  X0=1
  Relational Operator : RelationalOperator  Operator=~=  InputSameDT=on
  out_1 : Outport  InitialOutput=0
  wires:
  Relational Operator/1 -> out_1/1
  Memory/1 -> Relational Operator/1
  in_1/1 -> Relational Operator/2, Memory/1
